simulink model "a1_walking_GM"  (R2022b)
settings: Solver=VariableStepAuto  StartTime=0.0  StopTime=1  RelTol=1e-3
model workspace (MAT data in the model file):
  Period = 2
values from neighbouring files (symbols this model uses):
  m = 12    [MPC_Controller.m]    (also in QP_Controller.m; TASK1_rotating_mpc.m; TASK1_walking_backward_mpc.m; TASK1_walking_forward_mpc.m)
  N = 10    [MPC_Controller.m]
undefined symbols (not defined in the file or in its folder): X, Y, Z
libraries: sm_lib x188, nesl_utility x125
(part 6 of 6)

== matlab function a1_walking_GM/Convert Forces to Torque/Force to Torque ==
  data: F input; Tau_RR output; RR_ang_vec input; RL_ang_vec input; FL_ang_vec input; FR_ang_vec input; Tau_FR output; Tau_FL output; Tau_RL output
function [Tau_RR,Tau_FR,Tau_FL,Tau_RL]= fcn(F,RR_ang_vec,RL_ang_vec,FL_ang_vec,FR_ang_vec)
    % TODO - Convert forces to torques using the inverse jacobian
    % Get forces from the force vector 
    % NOTE - VERIFY THAT THESE ARE THE CORRECT VECTORS (I am unsure)
    F_FL = F(1:3);
    F_RL = F(4:6);
    F_FR = F(7:9);
    F_RR = F(10:12);

    l1=0.045; % hip length
    l2=0.2; % thigh length
    l3=0.2; % calf length
    

    %% Calculate the force for the RR leg - NOTE: The right legs have the
    % same jacobians
    q = RR_ang_vec; %
    leg = 4;
  
    if leg==1 || leg==3 % left leg has sideSign 1
        sideSign=1;
    else
        sideSign=-1; % right leg has sideSign -1
    end
    s1=sin(q(1)); % for hip joint
    s2=sin(q(2)); % for thigh joint
    s3=sin(q(3)); % for calf joint

    c1=cos(q(1)); % for hip joint
    c2=cos(q(2)); % for thigh joint
    c3=cos(q(3)); % for calf joint
    
    c23=c2*c3-s2*s3;
    s23=s2*c3+c2*s3;
    J = eye(3);
    J(1,1)=0;
    J(2,1)=-sideSign*l1*s1+l2*c2*c1+l3*c23*c1;
    J(3,1)=sideSign*l1*c1+l2*c2*s1+l3*c23*s1;
    
    J(1,2)=-l3*c23-l2*c2;
    J(2,2)=-l2*s2*s1-l3*s23*s1;
    J(3,2)=l2*s2*c1+l3*s23*c1;

    J(1,3)=-l3*c23;
    J(2,3)=-l3*s23*s1;
    J(3,3)=l3*s23*c1;
    
    inJ_R_RR = transpose(J);
    Tau_RR = -inJ_R_RR*F_RR;

  
    %% Calculate the force for the FR leg - NOTE: The right legs have the
    % same jacobians
    q = FR_ang_vec; %
    leg = 2;
  
    if leg==1 || leg==3 % left leg has sideSign 1
        sideSign=1;
    else
        sideSign=-1; % right leg has sideSign -1
    end
    s1=sin(q(1)); % for hip joint
    s2=sin(q(2)); % for thigh joint
    s3=sin(q(3)); % for calf joint

    c1=cos(q(1)); % for hip joint
    c2=cos(q(2)); % for thigh joint
    c3=cos(q(3)); % for calf joint
    
    c23=c2*c3-s2*s3;
    s23=s2*c3+c2*s3;

    J(1,1)=0;
    J(2,1)=-sideSign*l1*s1+l2*c2*c1+l3*c23*c1;
    J(3,1)=sideSign*l1*c1+l2*c2*s1+l3*c23*s1;
    
    J(1,2)=-l3*c23-l2*c2;
    J(2,2)=-l2*s2*s1-l3*s23*s1;
    J(3,2)=l2*s2*c1+l3*s23*c1;

    J(1,3)=-l3*c23;
    J(2,3)=-l3*s23*s1;
    J(3,3)=l3*s23*c1;

    inJ_R_FR = transpose(J);
    Tau_FR = -inJ_R_FR*F_FR;

    %% Calculate the force for the FL leg - NOTE: The right legs have the
    % same jacobians
    q = FL_ang_vec; %
    leg = 1;
  
    if leg==1 || leg==3 % left leg has sideSign 1
        sideSign=1;
    else
        sideSign=-1; % right leg has sideSign -1
    end
    s1=sin(q(1)); % for hip joint
    s2=sin(q(2)); % for thigh joint
    s3=sin(q(3)); % for calf joint

    c1=cos(q(1)); % for hip joint
    c2=cos(q(2)); % for thigh joint
    c3=cos(q(3)); % for calf joint
    
    c23=c2*c3-s2*s3;
    s23=s2*c3+c2*s3;

    J(1,1)=0;
    J(2,1)=-sideSign*l1*s1+l2*c2*c1+l3*c23*c1;
    J(3,1)=sideSign*l1*c1+l2*c2*s1+l3*c23*s1;
    
    J(1,2)=-l3*c23-l2*c2;
    J(2,2)=-l2*s2*s1-l3*s23*s1;
    J(3,2)=l2*s2*c1+l3*s23*c1;

    J(1,3)=-l3*c23;
    J(2,3)=-l3*s23*s1;
    J(3,3)=l3*s23*c1;

    inJ_R_FL = transpose(J);
    Tau_FL = -inJ_R_FL*F_FL;


    %% Calculate the force for the RL leg - NOTE: The right legs have the
    % same jacobians
    q = RL_ang_vec; %
    leg = 3;
  
    if leg==1 || leg==3 % left leg has sideSign 1
        sideSign=1;
    else
        sideSign=-1; % right leg has sideSign -1
    end
    s1=sin(q(1)); % for hip joint
    s2=sin(q(2)); % for thigh joint
    s3=sin(q(3)); % for calf joint

    c1=cos(q(1)); % for hip joint
    c2=cos(q(2)); % for thigh joint
    c3=cos(q(3)); % for calf joint
    
    c23=c2*c3-s2*s3;
    s23=s2*c3+c2*s3;

    J(1,1)=0;
    J(2,1)=-sideSign*l1*s1+l2*c2*c1+l3*c23*c1;
    J(3,1)=sideSign*l1*c1+l2*c2*s1+l3*c23*s1;
    
    J(1,2)=-l3*c23-l2*c2;
    J(2,2)=-l2*s2*s1-l3*s23*s1;
    J(3,2)=l2*s2*c1+l3*s23*c1;

    J(1,3)=-l3*c23;
    J(2,3)=-l3*s23*s1;
    J(3,3)=l3*s23*c1;

    inJ_R_RL = transpose(J);
    Tau_RL = -inJ_R_RL*F_RL;

== matlab function a1_walking_GM/Rigid Body Controller/Controller ==
  data: data input; u output
function u = fcn(data)
% % TODO - MAKE CONTROLLER ONLY RUN EVERY dt
r1 = data(13:15); %FL
r2 = data(16:18); %RL
r3 = data(19:21); %FR
r4 = data(22:24); %RR

m = 12;
Ib = diag([0.0168, 0.0565, 0.064]);
g = [0;0;-9.81]; 
p = [x;y;z];
R = reshape(Rot(4:12),[3,3]); dp = [x_dot;y_dot;z_dot];
wb = [wx;wy;wz];
mu = 0.5;
S = diag([2,2,10,1,2,1]); alpha = 0.01;
Kp_p = diag([30,30,400]); Kd_p = diag([10,10,50]); Kp_R = diag([10,10,10]); Kd_R = diag([5,5,5]);
rpy = [0,0,0];
Rd = eul2rotm(rpy);
ypr_e = rotm2eul(Rd*R');
p_d = [0;0;0.3];
rpy_e = [ypr_e(3);ypr_e(2);ypr_e(1);];
ddp_d = Kp_p*(p_d - p) + Kd_p*(-dp); dw_d = Kp_R*rpy_e + Kd_R*(-wb);
A = [eye(3), eye(3), eye(3), eye(3); Vec2Skewmat(r1),Vec2Skewmat(r2),Vec2Skewmat(r3),Vec2Skewmat(r4)];
b_d = [m*(ddp_d - g);R*(Ib*dw_d + cross(wb, Ib*wb))];
H = A'*S*A + alpha*eye(12); 
f = -2*b_d'*S*A;
Aqp_block = [1 0 -mu; 
            -1 0 -mu; 
             0 1 -mu;
            0 -1 -mu; 
            0 0 1;
            0 0 -1];
Aqp = blkdiag(Aqp_block,Aqp_block,Aqp_block,Aqp_block); 
bqp_block = [0;0;0;0;500;-10];
bqp = [bqp_block;bqp_block;bqp_block;bqp_block];
options = optimoptions('quadprog','Display','off'); 
u = quadprog(H,f,Aqp,bqp,[],[],[],[],[],options);

u = 0;
end

function S = Vec2Skewmat(a) 
S = [0 -a(3) a(2);
     a(3) 0 -a(1);
    -a(2) a(1) 0];
end

== matlab function a1_walking_GM/Rear Left Leg/Separate Torques ==
  data: torque_vector input; hip_torque output; thigh_torque output; calf_torque output
function [hip_torque, thigh_torque, calf_torque] = fcn(torque_vector)

hip_torque = torque_vector(1);
thigh_torque = torque_vector(2);
calf_torque = torque_vector(3);

== matlab function a1_walking_GM/Front Right Leg/Separate Torques ==
  data: torque_vector input; hip_torque output; thigh_torque output; calf_torque output
function [hip_torque, thigh_torque, calf_torque] = fcn(torque_vector)

hip_torque = torque_vector(1);
thigh_torque = torque_vector(2);
calf_torque = torque_vector(3);

== matlab function a1_walking_GM/Rear Right Leg/Separate Torques ==
  data: torque_vector input; hip_torque output; thigh_torque output; calf_torque output
function [hip_torque, thigh_torque, calf_torque] = fcn(torque_vector)

hip_torque = torque_vector(1);
thigh_torque = torque_vector(2);
calf_torque = torque_vector(3);

== matlab function a1_walking_GM/Front Left Leg/Separate Torques ==
  data: torque_vector input; hip_torque output; thigh_torque output; calf_torque output
function [hip_torque, thigh_torque, calf_torque] = fcn(torque_vector)

hip_torque = torque_vector(1);
thigh_torque = torque_vector(2);
calf_torque = torque_vector(3);
